simulink model "powersupply_nonlinear"  (R2015b)
settings: Solver=ode45  StartTime=0.0  StopTime=2  MaxStep=4e-7  MinStep=1e-8  RelTol=1e-3
values from neighbouring files (symbols this model uses):
  f_sw = 50e3    (= 50000)    [PowerSupplyScript.m]    (also in master_conv.m; master_conv2.m; matlab.mat)
  r_val = 1    [PowerSupplyScript.m]    (also in master_conv.m; master_conv2.m; matlab.mat)
libraries: powerlib x17, powerlib_meascontrol x1
settings Model: Creator=Akshay  LastModifiedBy=Akshay
settings SolverCC: ZeroCrossAlgorithm=Adaptive
settings DataIOCC: LimitDataPoints=off  SaveFormat=StructureWithTime
settings HardwareCC: ProdWordSize=32  ProdHWDeviceType=Specified

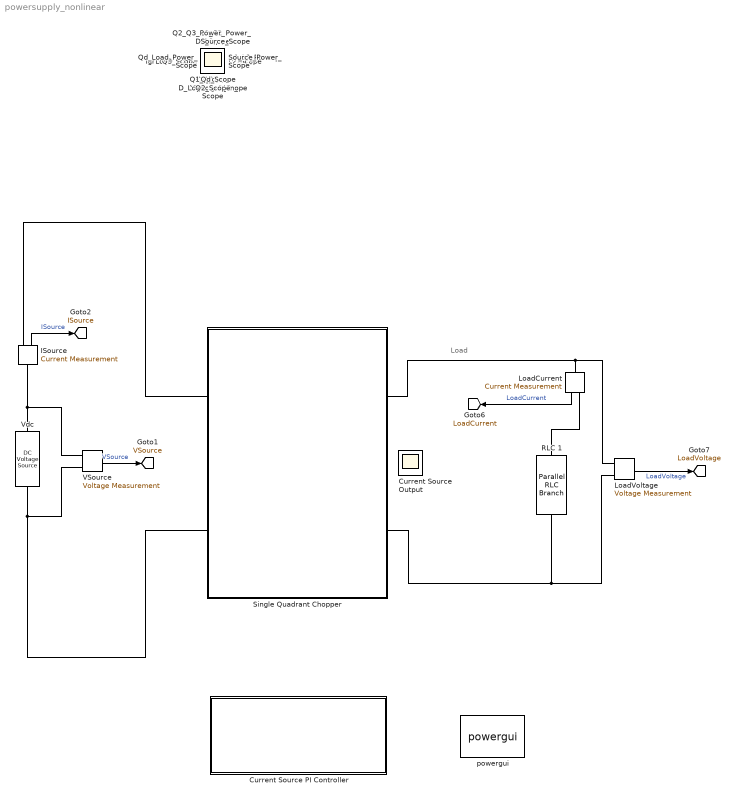
== system powersupply_nonlinear ==
  note: Load
  " RLC 1" : powerlib/Elements/Parallel RLC Branch  LConnTagsString=a  RConnTagsString=__new0  BranchType=R  Resistance=10  Inductance=1e-3  SetiL0=off  InitialCurrent=0  Capacitance=0.1e-6  Setx0=off  InitialVoltage=0  Measurements=None
  Current Source Output : Scope
      settings: Floating=on
  Current Source PI Controller : Subsystem
  ISource : powerlib/Measurements/Current Measurement  PhasorSimulation=off  OutputType=Complex  PSBequivalent=0
  LoadCurrent : powerlib/Measurements/Current Measurement  PhasorSimulation=off  OutputType=Complex  PSBequivalent=0
  LoadVoltage : powerlib/Measurements/Voltage Measurement  PhasorSimulation=off  OutputType=Complex  PSBequivalent=0
  Single Quadrant Chopper : Subsystem
  VSource : powerlib/Measurements/Voltage Measurement  PhasorSimulation=off  OutputType=Complex  PSBequivalent=0
  Vdc : powerlib/Electrical Sources/DC Voltage Source  Amplitude=100  Measurements=Voltage
  powergui : powerlib/powergui  Priority=1  SimulationMode=Continuous  SolverType=Backward Euler  SampleTime=0.01/f_sw  frequency=60  SPID=on  DisableSnubberDevices=off  DisableRonSwitches=off  DisableVfSwitches=off  SwTol=0  DisplayEquations=off  Interpol=off  ExternalGateDelay=off  methode=off  Ts=0  FunctionMessages=off  echomessages=off  HookPort=off  EnableUseOfTLC=off  x0status=zero  frequencyindice=0  Pbase=100e6  ErrMax=1e-4  Iterations=50  UnitsV=kV  UnitsW=MW  buscounter=0  RestoreLinks=warning  ResistiveCurrentMeasurement=off  Frange=[0:2:500]  Ylog=off  Xlog=on  ShowGrid=off  save=off  variable=ZData  structure=ScopeData  ZoomFFT=off  StartTime=0.0  cycles=5  DisplayStyle=2  fundamental=50  FreqAxis=off  MaxFrequency=50000  frequencyindicesteady=1  RmsSteady=1  display=off
  C2_Scope : Scope
  D1_Scope : Scope
  D_D1_Power_Scope : Scope
  D_Scope : Scope
  Ignition_Scope : Scope
  L1_C2_Power_Scope : Scope
  L1_Scope : Scope
  L2_Scope : Scope
  Load_Ignition_Scope : Scope
  Load_Scope : Scope
  Q1_L2_Power_Scope : Scope
  Q1_Scope : Scope
  Q2_Q3_Power_Scope : Scope
  Q2_Scope : Scope
  Q3_Scope : Scope
  Qd_Load_Power_Scope : Scope
  Qd_Scope : Scope
  Source_Power_Scope : Scope
  Source_Scope : Scope
  tag scope: ISource=global, LoadCurrent=global, LoadVoltage=global, VSource=global
  wires:
  LoadCurrent/1 -> [LoadCurrent]  "LoadCurrent"
  LoadVoltage/1 -> [LoadVoltage]  "LoadVoltage"
  VSource/1 -> [VSource]  "VSource"
  ISource/1 -> [ISource]  "ISource"
  connections:
  LoadCurrent/RConn1 -- " RLC 1"/LConn1
  LoadVoltage/LConn1 -- Single Quadrant Chopper/RConn1 -- LoadCurrent/LConn1
  ISource/RConn1 -- Single Quadrant Chopper/LConn1
  Single Quadrant Chopper/LConn2 -- VSource/LConn2 -- Vdc/LConn1
  LoadVoltage/LConn2 -- Single Quadrant Chopper/RConn2 -- " RLC 1"/RConn1
  ISource/LConn1 -- Vdc/RConn1 -- VSource/LConn1

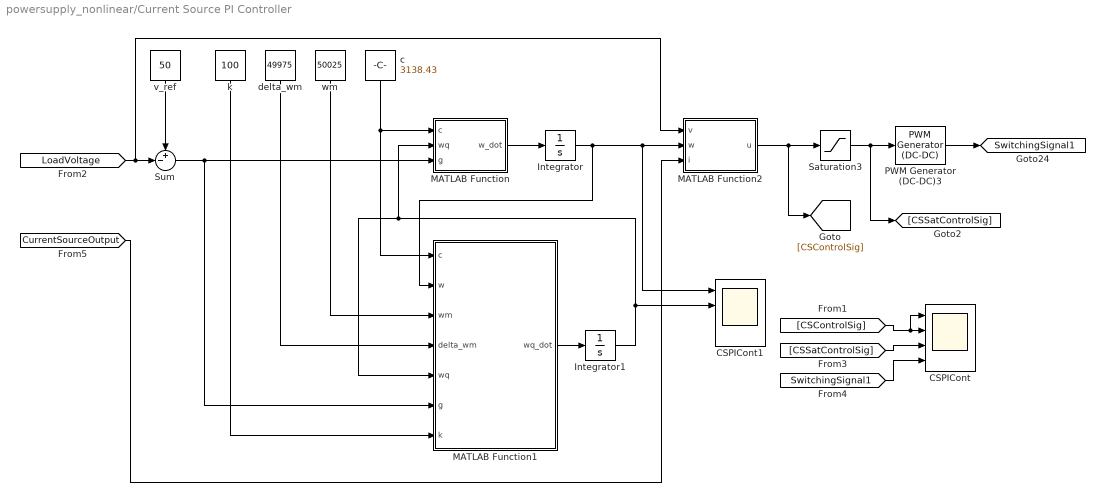
== system powersupply_nonlinear/Current Source PI Controller ==
  CSPICont : Scope  NumInputPorts=4
  CSPICont1 : Scope  NumInputPorts=4
  Integrator : Integrator  InitialCondition=50025
  Integrator1 : Integrator  InitialCondition=1
  MATLAB Function : MATLAB Function  TreatAsAtomicUnit=on
  MATLAB Function1 : MATLAB Function  TreatAsAtomicUnit=on
  MATLAB Function2 : MATLAB Function  TreatAsAtomicUnit=on
  PWM Generator (DC-DC)3 : powerlib_meascontrol/Pulse & Signal Generators/PWM Generator (DC-DC)  Fsw=20e3  Ts=0
  Saturation3 : Saturate  UpperLimit=0.99  LowerLimit=0
  Sum : Sum  Inputs=+-|
  c : Constant  Value=3138.43
  delta_wm : Constant  Value=49975
  k : Constant  Value=100
  v_ref : Constant  Value=50
  wm : Constant  Value=50025
  tag scope: SwitchingSignal1=global
  wires:
  Saturation3/1 -> [CSSatControlSig], PWM Generator (DC-DC)3/1
  PWM Generator (DC-DC)3/1 -> [SwitchingSignal1]
  [CSControlSig] -> CSPICont/1, CSPICont/2
  [CSSatControlSig] -> CSPICont/3
  [SwitchingSignal1] -> CSPICont/4
  MATLAB Function1/1(wq_dot) -> Integrator1/1
  MATLAB Function/1(w_dot) -> Integrator/1
  Integrator1/1 -> CSPICont1/2, MATLAB Function/2(wq), MATLAB Function1/5(wq)
  Integrator/1 -> MATLAB Function1/2(w), CSPICont1/1, MATLAB Function2/2(w)
  c/1 -> MATLAB Function/1(c), MATLAB Function1/1(c)
  wm/1 -> MATLAB Function1/3(wm)
  delta_wm/1 -> MATLAB Function1/4(delta_wm)
  k/1 -> MATLAB Function1/7(k)
  [LoadVoltage] -> MATLAB Function2/1(v), Sum/2
  v_ref/1 -> Sum/1
  Sum/1 -> MATLAB Function/3(g), MATLAB Function1/6(g)
  [CurrentSourceOutput] -> MATLAB Function2/3(i)
  MATLAB Function2/1(u) -> [CSControlSig], Saturation3/1

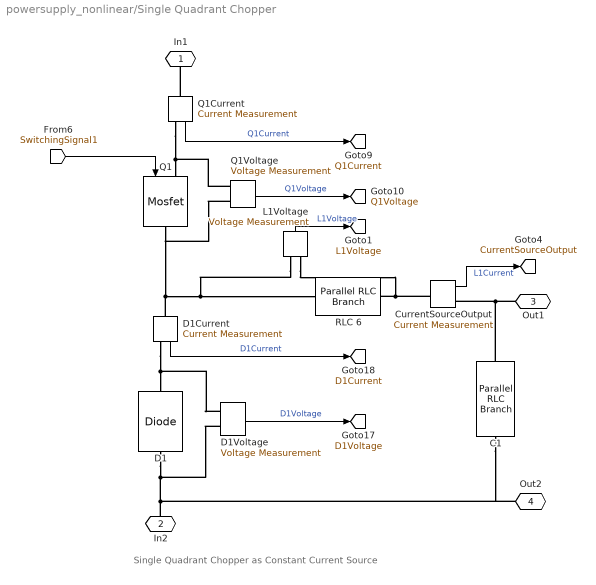
== system powersupply_nonlinear/Single Quadrant Chopper ==
  note: Single Quadrant Chopper as Constant Current Source
  " RLC 6" : powerlib/Elements/Parallel RLC Branch  LConnTagsString=a  RConnTagsString=__new0  BranchType=L  Resistance=50  Inductance=4e-3  SetiL0=off  InitialCurrent=100  Capacitance=0.3e-6  Setx0=off  InitialVoltage=0  Measurements=None
  C1 : powerlib/Elements/Parallel RLC Branch  LConnTagsString=a  RConnTagsString=__new0  BranchType=C  Resistance=r_val  Inductance=1e-3  SetiL0=off  InitialCurrent=0  Capacitance=100e-6  Setx0=off  InitialVoltage=0  Measurements=None
  CurrentSourceOutput : powerlib/Measurements/Current Measurement  PhasorSimulation=off  OutputType=Complex  PSBequivalent=0
  D1 : powerlib/Power Electronics/Diode  Ron=0.001  Lon=0  Vf=0.8  IC=0  UseSnubber=off  Rs=1e5  Cs=250e-9  Measurements=off
  D1Current : powerlib/Measurements/Current Measurement  PhasorSimulation=off  OutputType=Complex  PSBequivalent=0
  D1Voltage : powerlib/Measurements/Voltage Measurement  PhasorSimulation=off  OutputType=Complex  PSBequivalent=0
  "L1Voltage " : powerlib/Measurements/Voltage Measurement  PhasorSimulation=off  OutputType=Complex  PSBequivalent=0
  Q1 : powerlib/Power Electronics/Mosfet  Ron=0.1  Lon=0  Rd=0.01  Vfd=0  IC=0  Rs=1e5  Cs=inf  Measurements=off
  Q1Current : powerlib/Measurements/Current Measurement  PhasorSimulation=off  OutputType=Complex  PSBequivalent=0
  Q1Voltage : powerlib/Measurements/Voltage Measurement  PhasorSimulation=off  OutputType=Complex  PSBequivalent=0
  In1 : PMIOPort  Port=1  Side=Left
  In2 : PMIOPort  Port=2  Side=Left
  Out1 : PMIOPort  Port=3  Side=Right
  Out2 : PMIOPort  Port=4  Side=Right
  tag scope: CurrentSourceOutput=global, D1Current=global, D1Voltage=global, L1Voltage=global, Q1Current=global, Q1Voltage=global
  wires:
  CurrentSourceOutput/1 -> [CurrentSourceOutput]  "L1Current"
  [SwitchingSignal1] -> Q1/1
  Q1Current/1 -> [Q1Current]  "Q1Current"
  Q1Voltage/1 -> [Q1Voltage]  "Q1Voltage"
  D1Current/1 -> [D1Current]  "D1Current"
  D1Voltage/1 -> [D1Voltage]  "D1Voltage"
  "L1Voltage "/1 -> [L1Voltage]  "L1Voltage"
  connections:
  Q1Current/LConn1 -- In1/RConn1
  Q1Voltage/LConn2 -- Q1/RConn1 -- D1Current/LConn1 -- " RLC 6"/LConn1 -- "L1Voltage "/LConn1
  CurrentSourceOutput/LConn1 -- "L1Voltage "/LConn2 -- " RLC 6"/RConn1
  Q1Current/RConn1 -- Q1Voltage/LConn1 -- Q1/LConn1
  D1Current/RConn1 -- D1/RConn1 -- D1Voltage/LConn1
  D1Voltage/LConn2 -- C1/RConn1 -- Out2/RConn1 -- In2/RConn1 -- D1/LConn1
  Out1/RConn1 -- C1/LConn1 -- CurrentSourceOutput/RConn1

== matlab function powersupply_nonlinear/Current Source PI Controller/MATLAB Function1 ==
  data: wq_dot output; c input; w input; wm input; delta_wm input; wq input; g input; k input
function wq_dot = fcn(c,w,wm,delta_wm,wq,g,k)
wq_dot = c*(w-wm)*wq*g/delta_wm -k*((w-wm)^2/delta_wm^2-wq^2-1)*wq;

== matlab function powersupply_nonlinear/Current Source PI Controller/MATLAB Function ==
  data: w_dot output; c input; wq input; g input
function w_dot = fcn(c,wq,g)
w_dot = -c*wq^2*g;

== matlab function powersupply_nonlinear/Current Source PI Controller/MATLAB Function2 ==
  data: u output; v input; w input; i input
function u = fcn(v,w,i)
%u = 1/(1-v/(w*i));
u = (w*i)/v;
%u=w;
